simulink model "with_valve_dynamics"  (R2023b)
settings: Solver=ode1  StartTime=0.0  StopTime=0.30  FixedStep=1e-7  MaxStep=1e-6  RelTol=1e-6
InitFcn:
  | %% Parameters
  | 
  | param = struct();
  | 
  | % Volume of chambers
  | param.V1_0 = 1e-3;
  | param.V2_0 = 20e-6;
  | 
  | % Pressure rails
  | param.P_H = 20e6;
  | param.P_M = 10e6;
  | 
  | % Valve things
  | param.max_opening = 20e-3;
  | param.max_Avt = 0.5*0.25*pi*(param.max_opening)^2;
  | param.Cd = 0.6;
  | 
  | % Fluid properties
  | param.beta = 1.8e9;
  | param.rho = 870;
  | 
  | % Electric motor stuff
  | param.Kt = 70.5e-3;
  | param.Ke = 70.5e-3;
  | param.J_elec = 1530e-7;
  | 
  | % Pump things
  | param.J_hyd = 3000e-7;
  | param.hyd_D = 1.6e-6;    % In cc/rev
  | 
  | % Simulation time
  | T = 1;
  | param.on_time = 0;
  | 
  | % Linear Actuator Piston
  | param.Acap = 0.0045;
  | 
  | % Valve dynamics
  | param.wn = 50*2*pi;
  | param.zeta = 0.7;
settings Model: Creator=user  LastModifiedBy=user

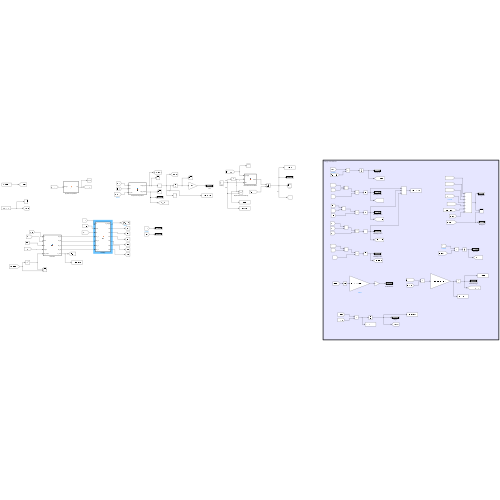
[thumbnail: Simulink's stored preview of the top-level diagram]
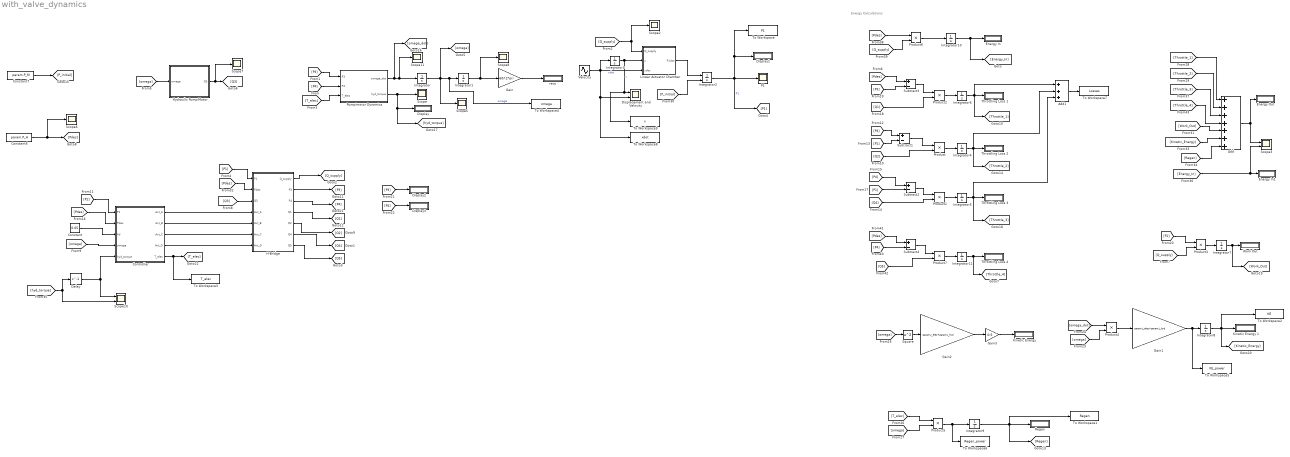
== system with_valve_dynamics ==
  note: Energy Calculations
  Add : Sum  Inputs=+++++++
  Add1 : Sum  Inputs=+++
  Constant : Constant  Value=0.05
  Constant6 : Constant  Value=param.P_H
  Constant7 : Constant  Value=param.P_M
  Controller : MATLAB Function  TreatAsAtomicUnit=on
  Delay : Delay  DelayLength=1
  Displacement and Velocity : Scope  NumInputPorts=2
  Display{,1..3} (4 alike) : Display
  Energy In : Display
  Energy In1 : Display
  Energy Out : Display
  Gain : Gain  Gain=60/(2*pi)
  Gain1 : Gain  Gain=param.J_elec+param.J_hyd
  Gain2 : Gain  Gain=param.J_elec+param.J_hyd
  Gain3 : Gain  Gain=0.5
  H-Bridge : MATLAB Function  TreatAsAtomicUnit=on
  Hydraulic Pump/Motor : MATLAB Function  TreatAsAtomicUnit=on
  Integrator{,1,3..11} (11 alike) : Integrator
  Integrator2 : Integrator  InitialConditionSource=external  InitialCondition=param.P_M
  Kinetic Energy : Display
  Kinetic Energy 1 : Display
  Linear Actuator Chamber : MATLAB Function  TreatAsAtomicUnit=on
  P1 : Scope
  Product{,1..7} (8 alike) : Product
  Pump/motor Dynamics : MATLAB Function  TreatAsAtomicUnit=on
  Regen : Display
  Scope{,2,5..8,11} (7 alike) : Scope
  Scope10 : Scope  NumInputPorts=2
  Scope3 : Scope  NumInputPorts=2
  Square : Math  Operator=square
  Subtract{1..4} (4 alike) : Sum  Inputs=+-
  Throttling Loss {1..4} (4 alike) : Display
  To Workspace : ToWorkspace  VariableName=P1  SaveFormat=Timeseries  SampleTime=-1
  To Workspace1 : ToWorkspace  VariableName=Regen  SaveFormat=Timeseries  SampleTime=-1
  To Workspace2 : ToWorkspace  VariableName=KE  SaveFormat=Timeseries  SampleTime=-1
  To Workspace3 : ToWorkspace  VariableName=T_elec  SaveFormat=Timeseries  SampleTime=-1
  To Workspace4 : ToWorkspace  VariableName=omega  SaveFormat=Timeseries  SampleTime=-1
  To Workspace5 : ToWorkspace  VariableName=KE_power  SaveFormat=Timeseries  SampleTime=-1
  To Workspace6 : ToWorkspace  VariableName=Regen_power  SaveFormat=Timeseries  SampleTime=-1
  To Workspace7 : ToWorkspace  VariableName=Losses  SaveFormat=Timeseries  SampleTime=-1
  To Workspace8 : ToWorkspace  VariableName=xdot  SaveFormat=Timeseries  SampleTime=-1
  To Workspace9 : ToWorkspace  VariableName=x  SaveFormat=Timeseries  SampleTime=-1
  Velocity : Sin  Amplitude=1e-2  Frequency=(2*pi)/0.3  Phase=pi/2  SampleTime=0
  Work Out : Display
  revs : Display
  wires:
  Pump/motor Dynamics/1(omega_dot) -> [omega_dot], Scope11/1, Integrator/1
  Integrator/1 -> Scope5/1, [omega], To Workspace4/1, Integrator1/1  "omega"
  Integrator1/1 -> Scope8/1, Gain/1
  Gain/1 -> revs/1
  Linear Actuator Chamber/1(P1dot) -> Integrator2/1
  Integrator2/1 -> [P1], To Workspace/1, Display1/1, P1/1  "P1"
  Constant/1 -> Controller/3(Kd)
  [P4] -> Pump/motor Dynamics/2(P4)
  [P3] -> Pump/motor Dynamics/1(P3)
  H-Bridge/1(Q_supply) -> [Q_supply]
  [Q_supply] -> Linear Actuator Chamber/1(Q_supply), Scope2/1
  [T_elec] -> Pump/motor Dynamics/3(T_elec)
  [P1] -> H-Bridge/1(P1)
  [Pdes] -> H-Bridge/2(Pdes)
  [omega] -> Hydraulic Pump/Motor/1(omega)
  Hydraulic Pump/Motor/1(Q3) -> Scope7/1, [Q3]
  [omega] -> Controller/4(omega)
  Pump/motor Dynamics/2(hyd_torque) -> [hyd_torque], Display/1, Scope/1
  [P_initial] -> Integrator2/2
  Constant7/1 -> [P_initial]
  Constant6/1 -> [Pdes], Scope6/1
  [hyd_torque] -> Scope10/2, Delay/1
  [Q3] -> H-Bridge/3(Q3)
  H-Bridge/2(P3) -> [P3]
  Velocity/1 -> Displacement and Velocity/2, To Workspace8/1, Linear Actuator Chamber/3(xdot), Integrator3/1  "xdot"
  Integrator3/1 -> Linear Actuator Chamber/2(x), To Workspace9/1, Displacement and Velocity/1  "x"
  [P3] -> Subtract1/1
  [P1] -> Subtract1/2
  [Q2] -> Product/2
  Subtract1/1 -> Product/1
  Product/1 -> Integrator4/1
  Integrator4/1 -> Add1/2, [Throttle_2], Throttling Loss 2/1
  Subtract2/1 -> Product1/1
  [Q4] -> Product1/2
  Product1/1 -> Integrator5/1
  Integrator5/1 -> Add1/3, [Throttle_3], Throttling Loss 3/1
  H-Bridge/5(Q2) -> [Q2]
  Subtract3/1 -> Product2/1
  [Q1] -> Product2/2
  Product2/1 -> Integrator6/1
  Integrator6/1 -> [Throttle_1], Add1/1, Throttling Loss 1/1
  [P1] -> Product3/1
  [Q_supply] -> Product3/2
  Product3/1 -> Integrator7/1
  Integrator7/1 -> [Work_Out], Work Out/1
  [P4] -> Display3/1
  [P3] -> Display2/1
  [omega_dot] -> Product4/1
  [omega] -> Product4/2
  Product4/1 -> Gain1/1
  Gain1/1 -> To Workspace5/1, Integrator8/1
  Integrator8/1 -> [Kinetic_Energy], To Workspace2/1, Kinetic Energy 1/1
  Gain2/1 -> Gain3/1
  [omega] -> Square/1
  Square/1 -> Gain2/1
  Gain3/1 -> Kinetic Energy/1
  [P1] -> Subtract2/2
  [P4] -> Subtract2/1
  H-Bridge/4(Q1) -> [Q1]
  [Pdes] -> Subtract3/1
  [P3] -> Subtract3/2
  [omega] -> Product5/2
  Integrator9/1 -> To Workspace1/1, [Regen], Regen/1
  Product5/1 -> To Workspace6/1, Integrator9/1
  [T_elec] -> Product5/1
  [Energy_In] -> Energy In1/1, Scope3/2
  Add/1 -> Energy Out/1, Scope3/1
  [Throttle_2] -> Add/2
  [Throttle_1] -> Add/1
  [Throttle_3] -> Add/3
  [Work_Out] -> Add/5
  [Kinetic_Energy] -> Add/6
  [Regen] -> Add/7
  Add1/1 -> To Workspace7/1
  [Pdes] -> Product6/1
  [Q_supply] -> Product6/2
  Product6/1 -> Integrator10/1
  Integrator10/1 -> [Energy_In], Energy In/1
  Delay/1 -> Scope10/1, Controller/5(hyd_torque)
  H-Bridge/3(P4) -> [P4]
  [P4] -> Subtract4/2
  [Pdes] -> Subtract4/1
  H-Bridge/6(Q4) -> [Q4]
  H-Bridge/7(Q5) -> [Q5]
  [Q5] -> Product7/2
  Subtract4/1 -> Product7/1
  Product7/1 -> Integrator11/1
  Integrator11/1 -> [Throttle_4], Throttling Loss 4/1
  [Throttle_4] -> Add/4
  [P1] -> Controller/1(P1)
  [Pdes] -> Controller/2(Pdes)
  Controller/1(Avt_A) -> H-Bridge/4(Avt_A)
  Controller/2(Avt_B) -> H-Bridge/5(Avt_B)
  Controller/3(Avt_C) -> H-Bridge/6(Avt_C)
  Controller/4(Avt_D) -> H-Bridge/7(Avt_D)
  Controller/5(T_elec) -> To Workspace3/1, [T_elec]

== matlab function with_valve_dynamics/Pump//motor Dynamics ==
  data: omega_dot output; P3 input; P4 input; param parameter; T_elec input; hyd_torque output
function [omega_dot, hyd_torque] = fcn(P3, P4, param, T_elec)

hyd_torque = (param.hyd_D/(2*pi))*(P3-P4);
omega_dot = (1/(param.J_elec+param.J_hyd))*(hyd_torque - T_elec);

== matlab function with_valve_dynamics/Hydraulic Pump//Motor ==
  data: Q3 output; omega input; param parameter
function Q3   = fcn(omega, param)

Q3 = (param.hyd_D/(2*pi))*omega;

== matlab function with_valve_dynamics/Controller ==
  data: P1 input; Avt_A output; Pdes input; Kd input; omega input; hyd_torque input; Avt_B output; Avt_C output; Avt_D output; T_elec output; param parameter
function [Avt_A, Avt_B, Avt_C, Avt_D, T_elec] = fcn(P1, Pdes, Kd, omega, hyd_torque, param)

if abs(P1-Pdes)<1e4 

    % Phase 2

    Avt_A = param.max_Avt;
    Avt_B = param.max_Avt;
    Avt_C = 0;
    Avt_D = param.max_Avt;

    if omega < 1
        T_elec = Kd*omega;
    else
        T_elec = 30;
    end

else

    % Phase 1

    Avt_A = param.max_Avt;
    Avt_B = 0;
    Avt_C = param.max_Avt;
    Avt_D = 0;

    if omega >= 300
        T_elec = hyd_torque;
    else
        T_elec = -30;
    end

end

== matlab function with_valve_dynamics/Linear Actuator Chamber ==
  data: P1dot output; Q_supply input; param parameter; x input; xdot input
function P1dot = fcn(Q_supply, param, x, xdot)

P1dot = (param.beta/(param.V1_0+param.Acap*x))*(Q_supply-param.Acap*xdot);

== matlab function with_valve_dynamics/H-Bridge ==
  data: P1 input; Pdes input; Q3 input; param parameter; Q_supply output; P3 output; P4 output; Q1 output; Avt_A input; Q2 output; Avt_B input; Avt_C input; Avt_D input; Q4 output; Q5 output
function [Q_supply, P3, P4, Q1, Q2, Q4, Q5] = fcn(P1, Pdes, Q3, param, Avt_A, Avt_B, Avt_C, Avt_D)

k_A = param.Cd*Avt_A*sqrt(2/param.rho);
k_B = param.Cd*Avt_B*sqrt(2/param.rho);
k_C = param.Cd*Avt_C*sqrt(2/param.rho);
k_D = param.Cd*Avt_D*sqrt(2/param.rho);

sigma1 = k_A^2 + k_B^2;
sigma2 = (Pdes-P1)*sigma1 - Q3^2;
sigma3 = k_C^2 + k_D^2;
sigma4 = (Pdes-P1)*sigma3 - Q3^2;

% Pressure on one side of the hyd motor
P3 = (P1*k_B^2 + Pdes*k_A^2 + Q3^2 - (2*Q3*k_A*(Q3*k_A + k_B*sqrt(abs(sigma2))*sign(sigma2)))/sigma1)/sigma1;

% Pressure on the other side of the hyd motor
P4 = (P1*k_C^2 + Pdes*k_D^2 + Q3^2 - (2*Q3*k_D*(Q3*k_D + k_C*sqrt(abs(sigma4))*sign(sigma4)))/sigma3)/sigma3;

% Flow through valve A
Q1 = k_A*sqrt(abs(Pdes-P3))*sign(Pdes-P3);

% Flow through valve B
Q2 = k_B*sqrt(abs(P3-P1))*sign(P3-P1);

% Flow through valve C
Q4 = k_C*sqrt(abs(P4-P1))*sign(P4-P1);

% Flow through valve D
Q5 = k_D*sqrt(abs(Pdes-P4))*sign(Pdes-P4);

% Supply going to the linear actuator chamber
Q_supply = Q2 + Q4;
